simulink model "Virtual_Second_Order_System"  (R2020b)
settings: Solver=ode4  StartTime=0.0  StopTime=20  FixedStep=0.01  RelTol=1e-3
settings Model: Creator=zxz  LastModifiedBy=zxz

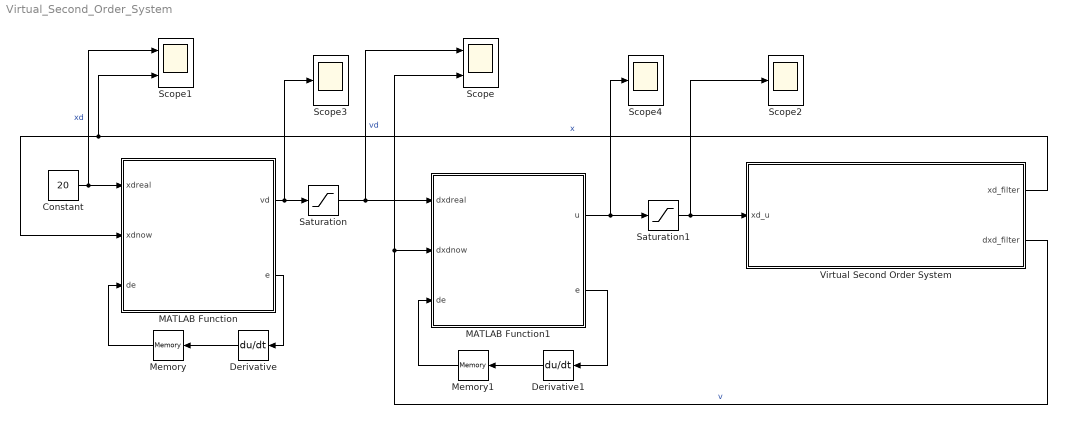
== system Virtual_Second_Order_System ==
  Constant : Constant  Value=20
  Derivative : Derivative
  Derivative1 : Derivative
  MATLAB Function : MATLAB Function  TreatAsAtomicUnit=on
  MATLAB Function1 : MATLAB Function  TreatAsAtomicUnit=on
  Memory : Memory
  Memory1 : Memory
  Saturation : Saturate  UpperLimit=2  LowerLimit=-2
  Saturation1 : Saturate  UpperLimit=1  LowerLimit=-1
  Scope : Scope  NumInputPorts=2
  Scope1 : Scope  NumInputPorts=2
  Scope2 : Scope
  Scope3 : Scope
  Scope4 : Scope
  Virtual Second Order System : Subsystem
  wires:
  MATLAB Function/2(e) -> Derivative/1
  Memory/1 -> MATLAB Function/3(de)
  Derivative/1 -> Memory/1
  Constant/1 -> Scope1/1, MATLAB Function/1(xdreal)  "xd"
  Virtual Second Order System/1(xd_filter) -> MATLAB Function/2(xdnow), Scope1/2  "x"
  MATLAB Function1/2(e) -> Derivative1/1
  Derivative1/1 -> Memory1/1
  Memory1/1 -> MATLAB Function1/3(de)
  Virtual Second Order System/2(dxd_filter) -> Scope/2, MATLAB Function1/2(dxdnow)  "v"
  MATLAB Function/1(vd) -> Scope3/1, Saturation/1
  Saturation/1 -> Scope/1, MATLAB Function1/1(dxdreal)  "vd"
  MATLAB Function1/1(u) -> Scope4/1, Saturation1/1
  Saturation1/1 -> Scope2/1, Virtual Second Order System/1(xd_u)

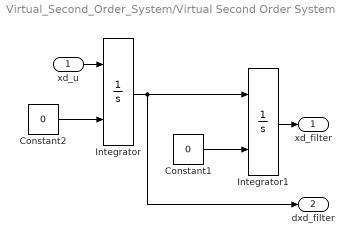
== system Virtual_Second_Order_System/Virtual Second Order System ==
  xd_u : Inport
  Constant1 : Constant  Value=0
  Constant2 : Constant  Value=0
  Integrator : Integrator  InitialConditionSource=external
  Integrator1 : Integrator  InitialConditionSource=external
  xd_filter : Outport
  dxd_filter : Outport  Port=2
  wires:
  Constant1/1 -> Integrator1/2
  Integrator/1 -> dxd_filter/1, Integrator1/1
  Constant2/1 -> Integrator/2
  xd_u/1 -> Integrator/1
  Integrator1/1 -> xd_filter/1

== matlab function Virtual_Second_Order_System/MATLAB Function1 ==
  data: dxdreal input; u output; dxdnow input; de input; e output
function [u,e] = Velocity_Control(dxdreal,dxdnow,de)
kp = 5;
kd = 0.1;

e=dxdreal-dxdnow;

u = kp*e+kd*de;

== matlab function Virtual_Second_Order_System/MATLAB Function ==
  data: xdreal input; vd output; xdnow input; de input; e output
function [vd,e] = Position_Control(xdreal,xdnow,de)
kp = 1;
kd = 0.1;

e=xdreal-xdnow;

vd = kp*e+kd*de;
